simulink model "pidcontroller"  (R2019b)
settings: Solver=VariableStepAuto  StartTime=0.0  StopTime=250  RelTol=1e-3
values from neighbouring files (symbols this model uses):
  x0 = [0, 0, 0.05, 2, 0, 0.01, 0.02, 0, 0, 0, 0, 0]    [createmodels.m]    (also in pidcontrolstartupscript.m = [0, 0, 0.05, 8, 0, 0.01, 0.02, 0, 0, 0, 0, 0])
undefined symbols (not defined in the file or in its folder): scalemodelstatefunction
libraries: simulink x2, aerolibanim x1
settings Model: SimulationMode=accelerator  Creator=Vlad  LastModifiedBy=Vlad

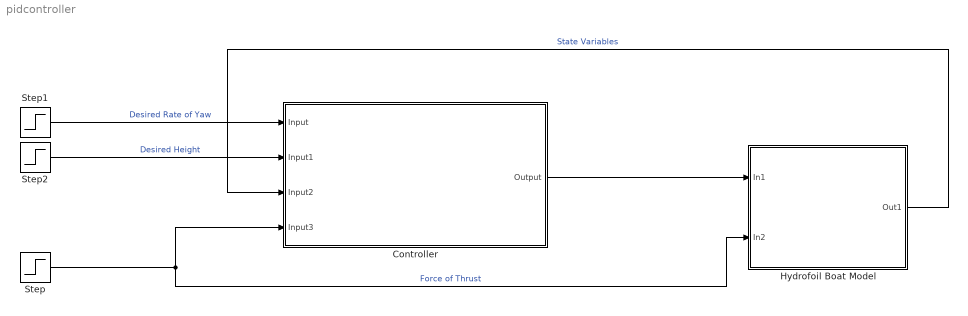
== system pidcontroller ==
  Controller : Subsystem
  Hydrofoil Boat Model : Subsystem
  Step : Step  Time=30  After=100  SampleTime=0
  Step1 : Step  Time=50  After=0.5  SampleTime=0
  Step2 : Step  Time=0  After=-0.5  SampleTime=0
  wires:
  Step/1 -> Controller/4(Input3), Hydrofoil Boat Model/2(In2)  "Force of Thrust"
  Step2/1 -> Controller/2(Input1)  "Desired Height"
  Controller/1(Output) -> Hydrofoil Boat Model/1(In1)
  Hydrofoil Boat Model/1(Out1) -> Controller/3(Input2)  "State Variables"
  Step1/1 -> Controller/1(Input)  "Desired Rate of Yaw"

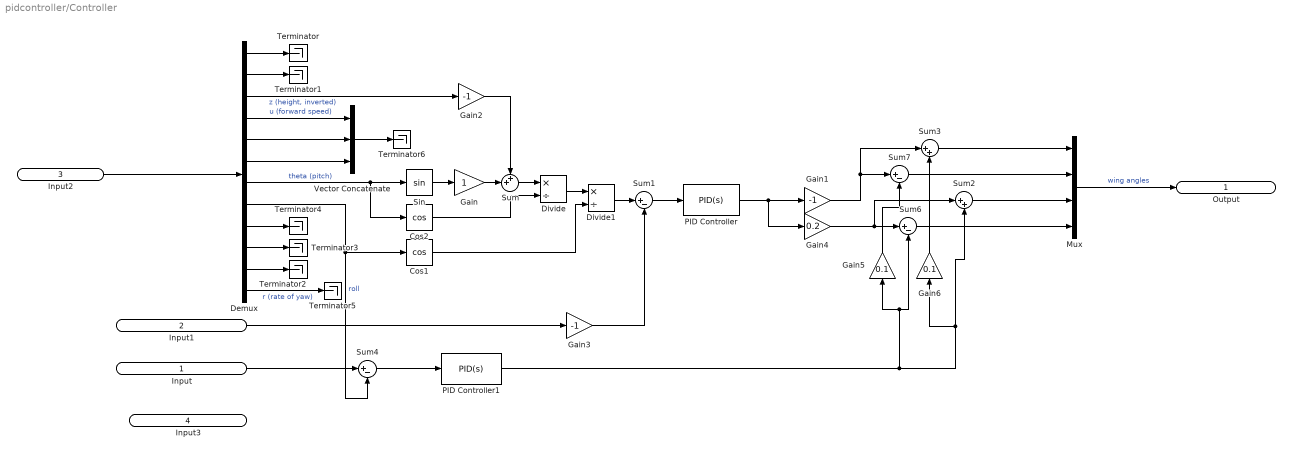
== system pidcontroller/Controller ==
  Input : Inport
  Input1 : Inport  Port=2
  Input2 : Inport  Port=3
  Input3 : Inport  Port=4
  Cos1 : Trigonometry  Operator=cos
  Cos2 : Trigonometry  Operator=cos
  Demux : Demux  Outputs=12
  Divide : Product  Inputs=*/
  Divide1 : Product  Inputs=*/
  Gain : Gain
  Gain1 : Gain  Gain=-1
  Gain2 : Gain  Gain=-1
  Gain3 : Gain  Gain=-1
  Gain4 : Gain  Gain=0.2
  Gain5 : Gain  Gain=0.1
  Gain6 : Gain  Gain=0.1
  Mux : Mux
  PID Controller : simulink/Continuous/PID Controller  Controller=PID  Form=Parallel  TimeDomain=Continuous-time  SampleTime=-1  IntegratorMethod=Forward Euler  FilterMethod=Forward Euler  ControllerParametersSource=internal  P=300  I=0.2  D=2000  UseFilter=on  N=100  TunerSelectOption=Transfer Function Based (PID Tuner App)  InitialConditionSource=internal  InitialConditionForIntegrator=0  InitialConditionForFilter=0  DifferentiatorICPrevScaledInput=0  ExternalReset=none  TrackingMode=off  Kt=1  LimitOutput=on  UpperSaturationLimit=15  LowerSaturationLimit=-5  LinearizeAsGain=on  AntiWindupMode=none  Kb=1  POutMin=[]  POutMax=[]  IOutMin=[]  IOutMax=[]  DOutMin=[]  DOutMax=[]  NOutMin=[]  NOutMax=[]  SumOutMin=[]  SumOutMax=[]  SaturationOutMin=[]  SaturationOutMax=[]  PParamMin=[]  PParamMax=[]  IParamMin=[]  IParamMax=[]  DParamMin=[]  DParamMax=[]  NParamMin=[]  NParamMax=[]  KbParamMin=[]  KbParamMax=[]  KtParamMin=[]  KtParamMax=[]  KbOutMin=[]  KbOutMax=[]  KtOutMin=[]  KtOutMax=[]  IntegratorOutMin=[]  IntegratorOutMax=[]  FilterOutMin=[]  FilterOutMax=[]  SumI1OutMin=[]  SumI1OutMax=[]  SumI2OutMin=[]  SumI2OutMax=[]  SumI3OutMin=[]  SumI3OutMax=[]  SumI4OutMin=[]  SumI4OutMax=[]  SumDOutMin=[]  SumDOutMax=[]  DifferentiatorOutMin=[]  DifferentiatorOutMax=[]  FilterDiffOutCoefMin=[]  FilterDiffOutCoefMax=[]  ReciprocalOutMin=[]  ReciprocalOutMax=[]  SumDenOutMin=[]  SumDenOutMax=[]  SumNumOutMin=[]  SumNumOutMax=[]  DivideOutMin=[]  DivideOutMax=[]  IntegratorContinuousStateAttributes=''  IntegratorStateMustResolveToSignalObject=off  IntegratorRTWStateStorageClass=Auto  FilterContinuousStateAttributes=''  FilterStateMustResolveToSignalObject=off  FilterRTWStateStorageClass=Auto  ParallelPVariant=InternalParameters  IdealPVariant=Disabled  IVariant=InternalParameters  DVariant=InternalParameters  IntegratorVariant=Continuous  SatVariant=Enabled  AWVariant=Passthrough  PCopyVariant=Disabled  TRVariant=Disabled  FdbkBlocksVariant=Forward  IdealPFdbkVariant=Disabled  SatFdbkVariant=Disabled  DerivativeFilterVariant=ContFilter  NVariant=InternalParameters  NCopyVariant=Disabled  FilterICVariant=InternalICsFilter  IntegratorICVariant=InternalICs  ExternalResetVariant=Disabled  TRSumVariant=Passthrough  SumFdbkVariant=Disabled  SumVariant=Sum_PID
  PID Controller1 : simulink/Continuous/PID Controller  Controller=PID  Form=Parallel  TimeDomain=Continuous-time  SampleTime=-1  IntegratorMethod=Forward Euler  FilterMethod=Forward Euler  ControllerParametersSource=internal  P=2  I=0.01  D=20  UseFilter=on  N=100  TunerSelectOption=Transfer Function Based (PID Tuner App)  InitialConditionSource=internal  InitialConditionForIntegrator=0  InitialConditionForFilter=0  DifferentiatorICPrevScaledInput=0  ExternalReset=none  TrackingMode=off  Kt=1  LimitOutput=on  UpperSaturationLimit=10  LowerSaturationLimit=-10  LinearizeAsGain=on  AntiWindupMode=none  Kb=1  POutMin=[]  POutMax=[]  IOutMin=[]  IOutMax=[]  DOutMin=[]  DOutMax=[]  NOutMin=[]  NOutMax=[]  SumOutMin=[]  SumOutMax=[]  SaturationOutMin=[]  SaturationOutMax=[]  PParamMin=[]  PParamMax=[]  IParamMin=[]  IParamMax=[]  DParamMin=[]  DParamMax=[]  NParamMin=[]  NParamMax=[]  KbParamMin=[]  KbParamMax=[]  KtParamMin=[]  KtParamMax=[]  KbOutMin=[]  KbOutMax=[]  KtOutMin=[]  KtOutMax=[]  IntegratorOutMin=[]  IntegratorOutMax=[]  FilterOutMin=[]  FilterOutMax=[]  SumI1OutMin=[]  SumI1OutMax=[]  SumI2OutMin=[]  SumI2OutMax=[]  SumI3OutMin=[]  SumI3OutMax=[]  SumI4OutMin=[]  SumI4OutMax=[]  SumDOutMin=[]  SumDOutMax=[]  DifferentiatorOutMin=[]  DifferentiatorOutMax=[]  FilterDiffOutCoefMin=[]  FilterDiffOutCoefMax=[]  ReciprocalOutMin=[]  ReciprocalOutMax=[]  SumDenOutMin=[]  SumDenOutMax=[]  SumNumOutMin=[]  SumNumOutMax=[]  DivideOutMin=[]  DivideOutMax=[]  IntegratorContinuousStateAttributes=''  IntegratorStateMustResolveToSignalObject=off  IntegratorRTWStateStorageClass=Auto  FilterContinuousStateAttributes=''  FilterStateMustResolveToSignalObject=off  FilterRTWStateStorageClass=Auto  ParallelPVariant=InternalParameters  IdealPVariant=Disabled  IVariant=InternalParameters  DVariant=InternalParameters  IntegratorVariant=Continuous  SatVariant=Enabled  AWVariant=Passthrough  PCopyVariant=Disabled  TRVariant=Disabled  FdbkBlocksVariant=Forward  IdealPFdbkVariant=Disabled  SatFdbkVariant=Disabled  DerivativeFilterVariant=ContFilter  NVariant=InternalParameters  NCopyVariant=Disabled  FilterICVariant=InternalICsFilter  IntegratorICVariant=InternalICs  ExternalResetVariant=Disabled  TRSumVariant=Passthrough  SumFdbkVariant=Disabled  SumVariant=Sum_PID
  Sin : Trigonometry
  Sum : Sum  Inputs=++|
  Sum{1,4,6..7} (4 alike) : Sum  Inputs=|+-
  Sum2 : Sum  Inputs=|++
  Sum3 : Sum  Inputs=|++
  Terminator{,1..6} (7 alike) : Terminator
  Vector Concatenate : Concatenate  NumInputs=3
  Output : Outport
  wires:
  Input2/1 -> Demux/1
  Mux/1 -> Output/1  "wing angles"
  Demux/7 -> Cos2/1, Sin/1  "theta (pitch)"
  PID Controller/1 -> Gain1/1, Gain4/1
  Demux/3 -> Gain2/1  "z (height, inverted)"
  Demux/1 -> Terminator/1
  Demux/2 -> Terminator1/1
  Demux/6 -> Vector Concatenate/3
  Demux/5 -> Vector Concatenate/2
  Demux/9 -> Terminator4/1
  Demux/10 -> Terminator3/1
  Demux/11 -> Terminator2/1
  Demux/4 -> Vector Concatenate/1  "u (forward speed)"
  Demux/8 -> Sum4/2, Cos1/1  "roll"
  Sin/1 -> Gain/1
  Gain/1 -> Sum/2
  Sum/1 -> Divide/1
  Cos2/1 -> Divide/2
  Divide/1 -> Divide1/1
  Cos1/1 -> Divide1/2
  Divide1/1 -> Sum1/1
  Input1/1 -> Gain3/1
  Sum1/1 -> PID Controller/1
  Gain1/1 -> Sum7/1, Sum3/1
  Gain3/1 -> Sum1/2
  Gain4/1 -> Sum2/1, Sum6/1
  Gain2/1 -> Sum/1
  Sum7/1 -> Mux/2
  Sum3/1 -> Mux/1
  Sum2/1 -> Mux/3
  Sum6/1 -> Mux/4
  Input/1 -> Sum4/1
  Sum4/1 -> PID Controller1/1
  PID Controller1/1 -> Sum2/2, Gain6/1, Sum6/2, Gain5/1
  Gain5/1 -> Sum7/2
  Gain6/1 -> Sum3/2
  Demux/12 -> Terminator5/1  "r (rate of yaw)"
  Vector Concatenate/1 -> Terminator6/1

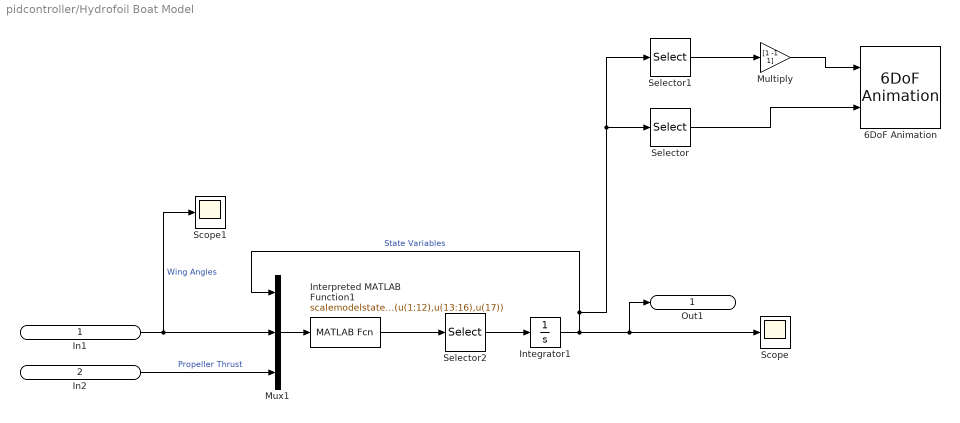
== system pidcontroller/Hydrofoil Boat Model ==
  In1 : Inport
  In2 : Inport  Port=2
  6DoF Animation : aerolibanim/6DoF Animation  u1=[0 30 -2 2 -1 0]  u2=0.1  u3=15  u4=[4000 0 -5000]  u5=Fixed position  u6=[20 20 -20]  u7=20  u8=off
      settings: SourceProductName=Aerospace Blockset
  Integrator1 : Integrator  InitialCondition=x0
  Interpreted MATLAB Function1 : MATLABFcn  MATLABFcn=scalemodelstatefunction(u(1:12),u(13:16),u(17))  OutputDimensions=12
  Multiply : Gain  Gain=[1 -1 1]
  Mux1 : Mux  Inputs=3
  Scope : Scope
  Scope1 : Scope
  Selector : Selector  InputPortWidth=12  IndexOptions=Index vector (dialog)  Indices=[8 7 9]  OutputSizes=1
  Selector1 : Selector  InputPortWidth=12  IndexOptions=Index vector (dialog)  Indices=[1 2 3]  OutputSizes=1
  Selector2 : Selector  InputPortWidth=12  IndexOptions=Index vector (dialog)  Indices=[1 2 3 4 5 6 7 8 9 10 11 12]  OutputSizes=1
  Out1 : Outport
  wires:
  Integrator1/1 -> Out1/1, Scope/1, Selector/1, Selector1/1, Mux1/1  "State Variables"
  Multiply/1 -> 6DoF Animation/1
  Selector1/1 -> Multiply/1
  Mux1/1 -> Interpreted MATLAB Function1/1
  Interpreted MATLAB Function1/1 -> Selector2/1
  Selector2/1 -> Integrator1/1
  Selector/1 -> 6DoF Animation/2
  In2/1 -> Mux1/3  "Propeller Thrust"
  In1/1 -> Scope1/1, Mux1/2  "Wing Angles"
